simulink model "audio_gain"  (R2020a)
settings: Solver=VariableStepAuto  StartTime=0.0  StopTime=32000/100e6  RelTol=1e-3
undefined symbols (not defined in the file): AXI4, Lite
libraries: xbsIndex_r4 x43
settings Model: Creator=ckb13136  LastModifiedBy=david
settings DataIOCC: ReturnWorkspaceOutputs=off
settings DebuggingCC: ArithmeticOperatorsInVariantConditions=warning
settings SFSimCC: SimUseLocalCustomCode=off  CustomCodeUndefinedFunction=UseInterfaceOnly
settings RTWCC: RTWUseLocalCustomCode=off

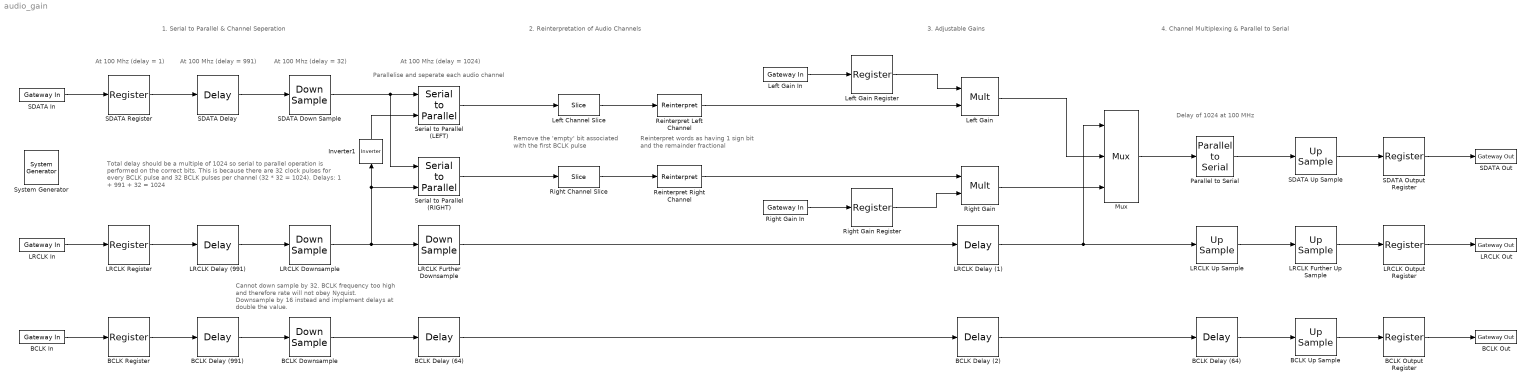
== system audio_gain ==
  note: 1. Serial to Parallel & Channel Seperation
  note: Reinterpret words as having 1 sign bit and the remainder fractional
  note: Parallelise and seperate each audio channel
  note: Remove the 'empty' bit associated with the first BCLK pulse
  note: At 100 Mhz (delay = 32)
  note: At 100 Mhz (delay = 1)
  note: Total delay should be a multiple of 1024 so serial to parallel operation
      | is performed on the correct bits. This is because there are 32 clock pulses
      | for every BCLK pulse and 32 BCLK pulses per channel (32 * 32 = 1024).
      | Delays: 1 + 991 + 32 = 1024
  note: Cannot down sample by 32. BCLK frequency too high and therefore rate will not obey Nyquist.
      | Downsample by 16 instead and implement delays at double the value.
  note: At 100 Mhz (delay = 1024)
  note: At 100 Mhz (delay = 991)
  note: 2. Reinterpretation of Audio Channels
  note: Delay of 1024 at 100 MHz
  note: 3. Adjustable Gains
  note: 4. Channel Multiplexing & Parallel to Serial
  " System Generator" : xbsIndex_r4/ System Generator  Tag=genX  xilinxfamily=zynq  part=xc7z020  speed=-1  package=clg400  synthesis_tool=Vivado  clock_wrapper=Clock Enables  directory=./netlist  proj_type=Vivado  Synth_file=Vivado Synthesis Defaults  Impl_file=Vivado Implementation Defaults  testbench=off  simulink_period=1/100e6  sysclk_period=10  dcm_input_clock_period=10  incr_netlist=off  trim_vbits=Everywhere in SubSystem  dbl_ovrd=According to Block Masks  core_generation=According to Block Masks  run_coregen=off  deprecated_control=off  eval_field=0  block_type=sysgen
  BCLK Delay (2) : xbsIndex_r4/Delay  rst=off  infoeditControl=Selection of Reset will increase slice count due to use of real FFs and instead of SRLs  en=off  latency=64  reg_retiming=off  dbl_ovrd=off  block_type=delay
  BCLK Delay (64) : xbsIndex_r4/Delay  rst=off  infoeditControl=Selection of Reset will increase slice count due to use of real FFs and instead of SRLs  en=off  latency=64  reg_retiming=off  dbl_ovrd=off  block_type=delay
  "BCLK Delay (64) " : xbsIndex_r4/Delay  rst=off  infoeditControl=Selection of Reset will increase slice count due to use of real FFs and instead of SRLs  en=off  latency=64  reg_retiming=off  dbl_ovrd=off  block_type=delay
  BCLK Delay (991) : xbsIndex_r4/Delay  rst=off  infoeditControl=Selection of Reset will increase slice count due to use of real FFs and instead of SRLs  en=off  latency=(32*32)-33  reg_retiming=off  dbl_ovrd=off  block_type=delay
  BCLK Downsample : xbsIndex_r4/Down Sample  sample_ratio=16  sample_phase="Last Value of Frame  (most efficient)"  en=off  rst=off  latency=2  dbl_ovrd=off  block_type=dsamp
  BCLK In : xbsIndex_r4/Gateway In  gui_display_data_type=Boolean  arith_type=Boolean  n_bits=1  bin_pt=0  preci_type=Single  exp_width=8  frac_width=24  rows=1  columns=1  quantization=Truncate  overflow=Saturate  period=1/100e6  UseAsADC=off  ADCChannel='1'  interface=None  automatic_assignment=off  address_offset=hex2dec('04')  intf_name=''  intf_description=''  default_value=0  timing_constraint=None  locs_specified=off  LOCs={}  io_standard={}  inherit_from_input=off  hdl_port=on  dbl_ovrd=off  block_type=gatewayin
  BCLK Out : xbsIndex_r4/Gateway Out  inherit_from_input=on  hdl_port=on  rows=1  columns=1  UseAsDAC=off  DACChannel='1'  interface=None  automatic_assignment=on  address_offset=hex2dec('00')  intf_name=''  intf_description=''  timing_constraint=None  locs_specified=off  LOCs={}  io_standard={}  block_type=gatewayout
  BCLK Output Register : xbsIndex_r4/Register  init=0  rst=off  en=off  dbl_ovrd=off  block_type=register
  BCLK Register : xbsIndex_r4/Register  init=0  rst=off  en=off  dbl_ovrd=off  block_type=register
  BCLK Up Sample : xbsIndex_r4/Up Sample  sample_ratio=16  copy_samples=on  en=off  latency=0  dbl_ovrd=off  block_type=usamp
  Inverter1 : xbsIndex_r4/Inverter  en=off  latency=0  dbl_ovrd=off  block_type=inv
  LRCLK Delay (1) : xbsIndex_r4/Delay  rst=off  infoeditControl=Selection of Reset will increase slice count due to use of real FFs and instead of SRLs  en=off  latency=1  reg_retiming=off  dbl_ovrd=off  block_type=delay
  LRCLK Delay (991) : xbsIndex_r4/Delay  rst=off  infoeditControl=Selection of Reset will increase slice count due to use of real FFs and instead of SRLs  en=off  latency=(32*32)-33  reg_retiming=off  dbl_ovrd=off  block_type=delay
  LRCLK Downsample : xbsIndex_r4/Down Sample  sample_ratio=32  sample_phase="Last Value of Frame  (most efficient)"  en=off  rst=off  latency=1  dbl_ovrd=off  block_type=dsamp
  LRCLK Further Downsample : xbsIndex_r4/Down Sample  sample_ratio=32  sample_phase="Last Value of Frame  (most efficient)"  en=off  rst=off  latency=1  dbl_ovrd=off  block_type=dsamp
  LRCLK Further Up Sample : xbsIndex_r4/Up Sample  sample_ratio=32  copy_samples=on  en=off  latency=0  dbl_ovrd=off  block_type=usamp
  LRCLK In : xbsIndex_r4/Gateway In  gui_display_data_type=Boolean  arith_type=Boolean  n_bits=1  bin_pt=0  preci_type=Single  exp_width=8  frac_width=24  rows=1  columns=1  quantization=Truncate  overflow=Saturate  period=1/100e6  UseAsADC=off  ADCChannel='1'  interface=None  automatic_assignment=off  address_offset=hex2dec('04')  intf_name=''  intf_description=''  default_value=0  timing_constraint=None  locs_specified=off  LOCs={}  io_standard={}  inherit_from_input=off  hdl_port=on  dbl_ovrd=off  block_type=gatewayin
  LRCLK Out : xbsIndex_r4/Gateway Out  inherit_from_input=on  hdl_port=on  rows=1  columns=1  UseAsDAC=off  DACChannel='1'  interface=None  automatic_assignment=on  address_offset=hex2dec('00')  intf_name=''  intf_description=''  timing_constraint=None  locs_specified=off  LOCs={}  io_standard={}  block_type=gatewayout
  LRCLK Output Register : xbsIndex_r4/Register  init=0  rst=off  en=off  dbl_ovrd=off  block_type=register
  LRCLK Register : xbsIndex_r4/Register  init=0  rst=off  en=off  dbl_ovrd=off  block_type=register
  LRCLK Up Sample : xbsIndex_r4/Up Sample  sample_ratio=32  copy_samples=on  en=off  latency=1  dbl_ovrd=off  block_type=usamp
  Left Channel Slice : xbsIndex_r4/Slice  nbits=31  boolean_output=off  mode=Upper Bit Location + Width  bit1=-1  base1=MSB of Input  bit0=0  base0=LSB of Input  dbl_ovrd=off  block_type=slice
  Left Gain : xbsIndex_r4/Mult  precision=User Defined  arith_type="Signed  (2's comp)"  n_bits=32  bin_pt=31  quantization=Truncate  overflow=Saturate  en=off  latency=1  use_behavioral_HDL=off  opt=Speed  use_embedded=on  optimum_pipeline=off  pipeline=on  dbl_ovrd=off  use_rpm=on  placement_style=Triangular  block_type=mult
  Left Gain In : xbsIndex_r4/Gateway In  gui_display_data_type=Fixed-point  arith_type=Unsigned  n_bits=4  bin_pt=3  preci_type=Single  exp_width=8  frac_width=24  rows=1  columns=1  quantization=Truncate  overflow=Saturate  period=(32*32)/100e6  UseAsADC=off  ADCChannel='1'  interface=AXI4-Lite  automatic_assignment=off  address_offset=hex2dec('00')  intf_name=''  intf_description=''  default_value=0  timing_constraint=None  locs_specified=off  LOCs={}  io_standard={}  inherit_from_input=off  hdl_port=on  dbl_ovrd=off  block_type=gatewayin
  Left Gain Register : xbsIndex_r4/Register  init=0  rst=off  en=off  dbl_ovrd=off  block_type=register
  Mux : xbsIndex_r4/Mux  inputs=2  en=off  latency=0  precision=User Defined  arith_type="Signed  (2's comp)"  n_bits=32  bin_pt=31  quantization=Truncate  overflow=Saturate  dbl_ovrd=off  block_type=mux
  Parallel to Serial : xbsIndex_r4/Parallel to Serial  output_order=Most Significant Word First  arith_type=Unsigned  output_bits=1  bin_pt=0  rst=off  en=off  latency=32  dbl_ovrd=off  block_type=p2s
      settings: infoedit=Each sample presented at the input becomes several samples presented serially at the output.
  Reinterpret Left Channel : xbsIndex_r4/Reinterpret  force_arith_type=on  arith_type="Signed  (2's comp)"  force_bin_pt=on  bin_pt=30  block_type=reinterpret
  Reinterpret Right Channel : xbsIndex_r4/Reinterpret  force_arith_type=on  arith_type="Signed  (2's comp)"  force_bin_pt=on  bin_pt=30  block_type=reinterpret
  Right Channel Slice : xbsIndex_r4/Slice  nbits=31  boolean_output=off  mode=Upper Bit Location + Width  bit1=-1  base1=MSB of Input  bit0=0  base0=LSB of Input  dbl_ovrd=off  block_type=slice
  Right Gain : xbsIndex_r4/Mult  precision=User Defined  arith_type="Signed  (2's comp)"  n_bits=32  bin_pt=31  quantization=Truncate  overflow=Saturate  en=off  latency=1  use_behavioral_HDL=off  opt=Speed  use_embedded=on  optimum_pipeline=off  pipeline=on  dbl_ovrd=off  use_rpm=on  placement_style=Triangular  block_type=mult
  Right Gain In : xbsIndex_r4/Gateway In  gui_display_data_type=Fixed-point  arith_type=Unsigned  n_bits=4  bin_pt=3  preci_type=Single  exp_width=8  frac_width=24  rows=1  columns=1  quantization=Truncate  overflow=Saturate  period=(32*32)/100e6  UseAsADC=off  ADCChannel='1'  interface=AXI4-Lite  automatic_assignment=off  address_offset=hex2dec('04')  intf_name=''  intf_description=''  default_value=0  timing_constraint=None  locs_specified=off  LOCs={}  io_standard={}  inherit_from_input=off  hdl_port=on  dbl_ovrd=off  block_type=gatewayin
  Right Gain Register : xbsIndex_r4/Register  init=0  rst=off  en=off  dbl_ovrd=off  block_type=register
  SDATA Delay : xbsIndex_r4/Delay  rst=off  infoeditControl=Selection of Reset will increase slice count due to use of real FFs and instead of SRLs  en=off  latency=(32*32)-33  reg_retiming=off  dbl_ovrd=off  block_type=delay
  SDATA Down Sample : xbsIndex_r4/Down Sample  sample_ratio=32  sample_phase="Last Value of Frame  (most efficient)"  en=off  rst=off  latency=1  dbl_ovrd=off  block_type=dsamp
  SDATA In : xbsIndex_r4/Gateway In  gui_display_data_type=Fixed-point  arith_type=Unsigned  n_bits=1  bin_pt=0  preci_type=Single  exp_width=8  frac_width=24  rows=1  columns=1  quantization=Truncate  overflow=Saturate  period=1/100e6  UseAsADC=off  ADCChannel='1'  interface=None  automatic_assignment=on  address_offset=hex2dec('00')  intf_name=''  intf_description=''  default_value=0  timing_constraint=None  locs_specified=off  LOCs={}  io_standard={}  inherit_from_input=off  hdl_port=on  dbl_ovrd=off  block_type=gatewayin
  SDATA Out : xbsIndex_r4/Gateway Out  inherit_from_input=on  hdl_port=on  rows=1  columns=1  UseAsDAC=off  DACChannel='1'  interface=None  automatic_assignment=on  address_offset=hex2dec('00')  intf_name=''  intf_description=''  timing_constraint=None  locs_specified=off  LOCs={}  io_standard={}  block_type=gatewayout
  SDATA Output Register : xbsIndex_r4/Register  init=0  rst=off  en=off  dbl_ovrd=off  block_type=register
  SDATA Register : xbsIndex_r4/Register  init=0  rst=off  en=off  dbl_ovrd=off  block_type=register
  SDATA Up Sample : xbsIndex_r4/Up Sample  sample_ratio=32  copy_samples=on  en=off  latency=0  dbl_ovrd=off  block_type=usamp
  Serial to Parallel (LEFT) : xbsIndex_r4/Serial to Parallel  input_order=Most Significant Word First  arith_type=Unsigned  output_bits=32  bin_pt=0  rst=off  en=on  latency=1  dbl_ovrd=off  block_type=s2p
      settings: infoedit=Groups of samples presented serially at the input become single samples presented at the output.
  Serial to Parallel (RIGHT) : xbsIndex_r4/Serial to Parallel  input_order=Most Significant Word First  arith_type=Unsigned  output_bits=32  bin_pt=0  rst=off  en=on  latency=1  dbl_ovrd=off  block_type=s2p
      settings: infoedit=Groups of samples presented serially at the input become single samples presented at the output.
  wires:
  SDATA In/1 -> SDATA Register/1
  LRCLK In/1 -> LRCLK Register/1
  BCLK In/1 -> BCLK Register/1
  BCLK Delay (991)/1 -> BCLK Downsample/1
  SDATA Delay/1 -> SDATA Down Sample/1
  SDATA Register/1 -> SDATA Delay/1
  LRCLK Downsample/1 -> LRCLK Further Downsample/1, Serial to Parallel (RIGHT)/2, Inverter1/1
  Serial to Parallel (RIGHT)/1 -> Right Channel Slice/1
  Left Channel Slice/1 -> Reinterpret Left Channel/1
  Right Channel Slice/1 -> Reinterpret Right Channel/1
  Serial to Parallel (LEFT)/1 -> Left Channel Slice/1
  LRCLK Delay (991)/1 -> LRCLK Downsample/1
  BCLK Downsample/1 -> BCLK Delay (64)/1
  BCLK Register/1 -> BCLK Delay (991)/1
  Inverter1/1 -> Serial to Parallel (LEFT)/2
  LRCLK Register/1 -> LRCLK Delay (991)/1
  SDATA Down Sample/1 -> Serial to Parallel (RIGHT)/1, Serial to Parallel (LEFT)/1
  LRCLK Further Downsample/1 -> LRCLK Delay (1)/1
  BCLK Delay (64)/1 -> BCLK Delay (2)/1
  Reinterpret Left Channel/1 -> Left Gain/2
  Reinterpret Right Channel/1 -> Right Gain/1
  Left Gain In/1 -> Left Gain Register/1
  Left Gain Register/1 -> Left Gain/1
  Right Gain In/1 -> Right Gain Register/1
  Right Gain Register/1 -> Right Gain/2
  BCLK Output Register/1 -> BCLK Out/1
  LRCLK Output Register/1 -> LRCLK Out/1
  SDATA Output Register/1 -> SDATA Out/1
  Parallel to Serial/1 -> SDATA Up Sample/1
  LRCLK Further Up Sample/1 -> LRCLK Output Register/1
  BCLK Delay (2)/1 -> "BCLK Delay (64) "/1
  LRCLK Up Sample/1 -> LRCLK Further Up Sample/1
  "BCLK Delay (64) "/1 -> BCLK Up Sample/1
  LRCLK Delay (1)/1 -> Mux/1, LRCLK Up Sample/1
  Right Gain/1 -> Mux/3
  Left Gain/1 -> Mux/2
  Mux/1 -> Parallel to Serial/1
  SDATA Up Sample/1 -> SDATA Output Register/1
  BCLK Up Sample/1 -> BCLK Output Register/1
